simulink model "DR_District_Resource_Planner_v2"  (R2026a)
settings: Solver=VariableStepAuto  StopTime=28800
undefined symbols (not defined in the file or in its folder): m, n
settings Model: Creator=Appasaheb  LastModifiedBy=Appasaheb

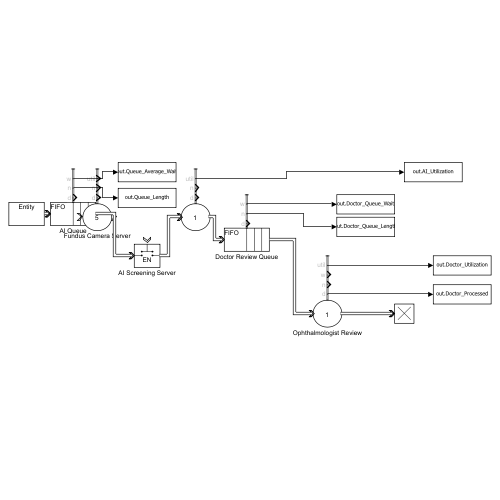
[thumbnail: Simulink's stored preview of the top-level diagram]
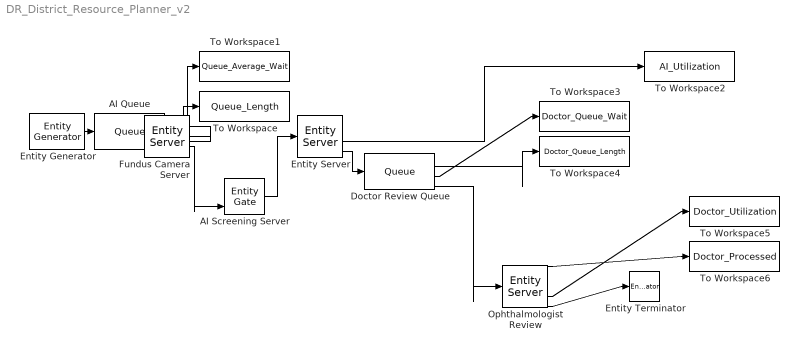
== system DR_District_Resource_Planner_v2 ==
  AI Queue : Queue  InputPortMessageModes=m  OutputPortMessageModes=n,n,n,m  NumberEntitiesDeparted=on  NumberEntitiesInBlock=on  AverageWait=on
      settings: OutputPortMap=o0,o1,o2,o5
  AI Screening Server : EntityGate  InputPortMessageModes=m,m  OutputPortMessageModes=m  OpenGateAtSimulationStart=on
  Doctor Review Queue : Queue  InputPortMessageModes=m  OutputPortMessageModes=n,n,n,m  NumberEntitiesDeparted=on  NumberEntitiesInBlock=on  AverageWait=on
      settings: OutputPortMap=o0,o1,o2,o5
  Entity Generator : EntityGenerator  OutputPortMessageModes=m  Period=28.8  EntityType=Structured  EntityTypeName=Entity
  Entity Server : EntityServer  InputPortMessageModes=m  OutputPortMessageModes=n,n,n,m  Capacity=1  ServiceTimeValue=8.56  NumberEntitiesDeparted=on  NumberEntitiesInBlock=on  Utilization=on
      settings: OutputPortMap=o0,o1,o5,o9
  Entity Terminator : EntityTerminator  InputPortMessageModes=m
  Fundus Camera Server : EntityServer  InputPortMessageModes=m  OutputPortMessageModes=n,n,n,m  ServiceTimeValue=240  NumberEntitiesDeparted=on  NumberEntitiesInBlock=on  Utilization=on
      settings: OutputPortMap=o0,o1,o5,o9
  Ophthalmologist Review : EntityServer  InputPortMessageModes=m  OutputPortMessageModes=n,n,n,n,m  Capacity=1  ServiceTimeValue=120  NumberEntitiesDeparted=on  NumberEntitiesInBlock=on  AverageWait=on  Utilization=on
      settings: OutputPortMap=o0,o1,o4,o5,o9
  To Workspace : ToWorkspace  VariableName=Queue_Length  SaveFormat=Timeseries  SampleTime=-1
  To Workspace1 : ToWorkspace  VariableName=Queue_Average_Wait  SaveFormat=Timeseries  SampleTime=-1
  To Workspace2 : ToWorkspace  VariableName=AI_Utilization  SaveFormat=Timeseries  SampleTime=-1
  To Workspace3 : ToWorkspace  VariableName=Doctor_Queue_Wait  SaveFormat=Timeseries  SampleTime=-1
  To Workspace4 : ToWorkspace  VariableName=Doctor_Queue_Length  SaveFormat=Timeseries  SampleTime=-1
  To Workspace5 : ToWorkspace  VariableName=Doctor_Utilization  SaveFormat=Timeseries  SampleTime=-1
  To Workspace6 : ToWorkspace  VariableName=Doctor_Processed  SaveFormat=Timeseries  SampleTime=-1
  wires:
  Entity Server/4 -> Doctor Review Queue/1
  Entity Generator/1 -> AI Queue/1
  AI Queue/4 -> AI Screening Server/2
  AI Queue/3 -> To Workspace1/1
  AI Queue/2 -> To Workspace/1
  Entity Server/3 -> To Workspace2/1
  Doctor Review Queue/4 -> Ophthalmologist Review/1
  Ophthalmologist Review/5 -> Entity Terminator/1
  Doctor Review Queue/3 -> To Workspace3/1
  Doctor Review Queue/2 -> To Workspace4/1
  Ophthalmologist Review/4 -> To Workspace5/1
  Ophthalmologist Review/1 -> To Workspace6/1
  AI Screening Server/1 -> Entity Server/1
